simulink library "renewableCustom_lib"  (R2025b)
settings: Solver=VariableStepAuto  StartTime=0.0  StopTime=10.0  RelTol=1e-3
undefined symbols (not defined in the file or in its folder): alpha, Base, D, Kd, Kp, Kt, Ld, Lq, PVController, PVInverter, Rs, T, Ts
libraries: slpidlib x2, eeTransforms x2, simulink x2
settings Model: Creator=rajarshd  LastModifiedBy=rajarshd

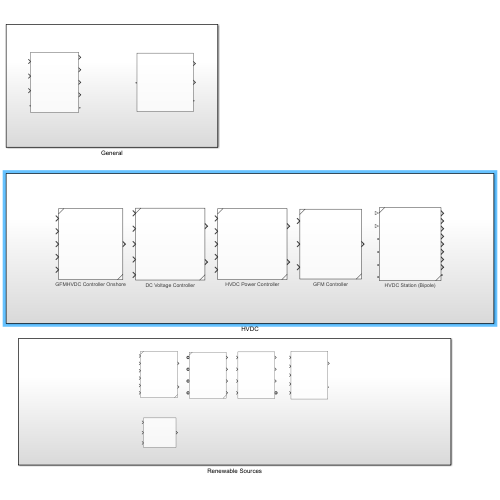
[thumbnail: Simulink's stored preview of the top-level diagram]
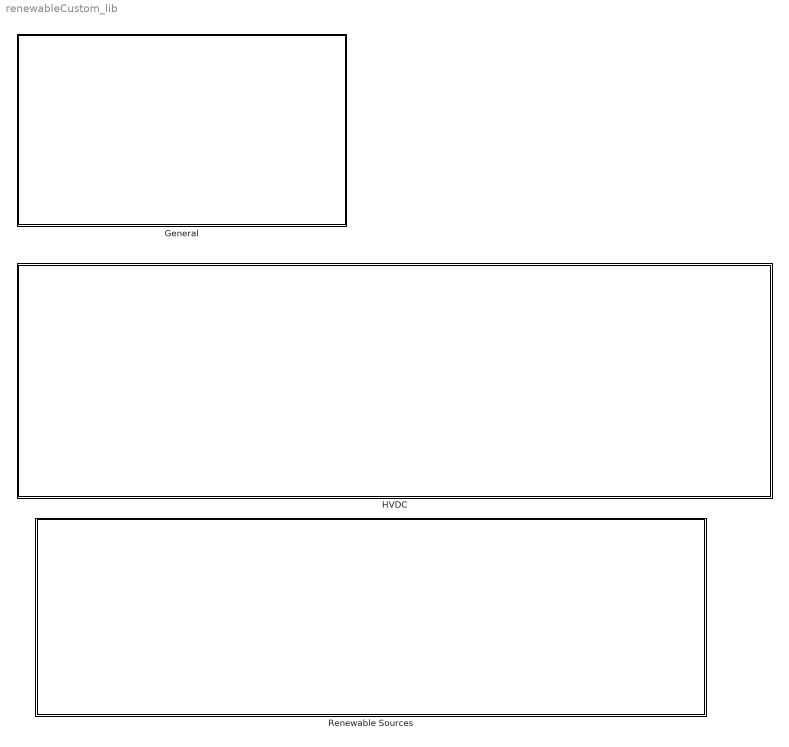
== system renewableCustom_lib ==
  General : Subsystem
  HVDC : Subsystem
  Renewable Sources : Subsystem

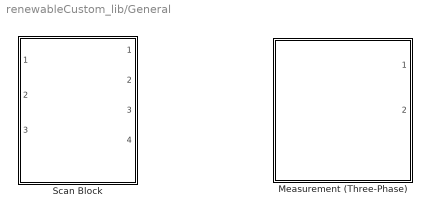
== system renewableCustom_lib/General ==
  Measurement (Three-Phase) : Subsystem  ReferencedSubsystem=MeasurementPLL  f=60  MVA=100e6  baseV=230e3
  Scan Block : Subsystem  ReferencedSubsystem=ScanBlockwithDC  F0=grid.frequency  Theta0=0  Kp_LF=100  Ki_LF=2000  Ts=5e-5  voltage=4.16e3  voltagedc=0  mva=0  Amplitude=0.01  Amplitude1=0  Amplitudedc=0  f=1:1:1e3  T=T  Tdis=5  Tend=10  VSelect=Equivalent Series Voltage (V)  Hold=Yes

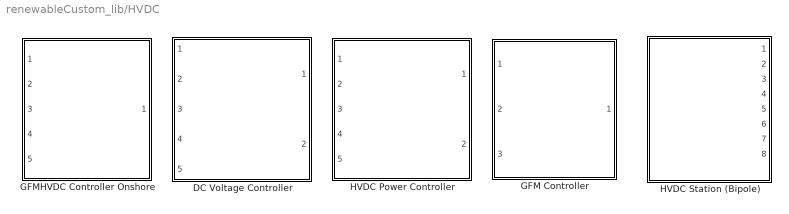
== system renewableCustom_lib/HVDC ==
  DC Voltage Controller : Subsystem  ReferencedSubsystem=DCVoltageControl  Kppll=100  Kipll=2000  frequency=60  initialPhase=0  sampleTime=-1  Kpicd=1.5  Kiicd=250  Kdicd=0  Kpicq=2  Kiicq=300  Kdicq=0  Kpv=20  Kiv=1  Kdv=0  L=5e-3  iMax=1.2  zBase=1.1  mVAbase=100e6  VdcBase=400e3
  GFM Controller : Subsystem  ReferencedSubsystem=WFController  Kpv=0  Kiv=0  Kpicd=0  Kiicd=0  Kpicq=0  Kiicq=0  mVAbase=0  frequency=0  zBase=0  iMax=0  L=0  Kv=0
  GFMHVDC Controller Onshore : Subsystem  ReferencedSubsystem=GFMHVDCControllerOnshore  D=10  J=0  frequency1=60  Pref=0  kc=0  Kq=0.1  VdRef=0  Imax1=1.2  l=5e-3  Kpv=5  Kiv=1  Vdc=0  Kpi=1.5  Kii=250
  HVDC Power Controller : Subsystem  ReferencedSubsystem=HVDCPowerControl  Kppll=PLL.Kp_pll  Kipll=PLL.Ki_pll  frequency=Grid.frequency  initialPhase=0  sampleTime=-1  Kpicd=PVController.Kp_ic  Kiicd=PVController.Ki_ic  Kdicd=0  Kpicq=PVController.Kp_ic  Kiicq=PVController.Ki_ic  Kdicq=0  Kpv=3.5  Kiv=10  Kdv=0.0  L=PVInverter.L*10  iMax=PVInverter.I_max_pu  zBase=Base.z_base  mVAbase=Base.MVA_base_new  VdcBase=PVController.Vdc_base
  HVDC Station (Bipole) : Subsystem  ReferencedSubsystem=HVDCSTATION  c=0  vc=0  L=0  VRated=0  SRated=0  t=0  Ts=0

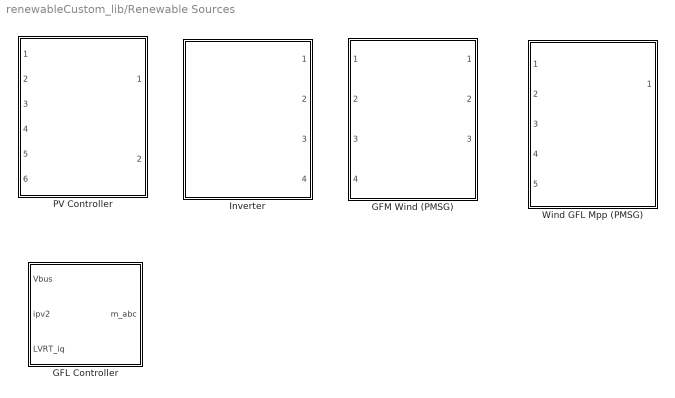
== system renewableCustom_lib/Renewable Sources ==
  GFL Controller : Subsystem  mask{Vref=1, fref=60, Pref=3e6, Qref=1e4, mp=1e-2, mv=2, P=Real power, MVA=5e7, zbase=2, L=3e-3, Imax=1.2, Td=3e-3, Kpic=2, Kiic=250, Kd=PVController.Kd}
      mask prompts: Vref "Voltage reference (PU)"; fref "Frequency reference (Hz)"; Pref "Real power reference (PU)"; Qref "Reactive power reference (PU)"; mp "Real power droop cofficient"; mv "Reactive power droop cofficient"; P "Priority mode"; MVA "Base Power (V*A)"; zbase "Base Impedance (Ohm)"; L "Filter Inductance (H)"; Imax "Inverter current limit (pu)"; Td "Sensor time delay (s)"; Kpic "Proportional gain"; Kiic "Integral gain"; Kd "Derevative gain"
      mask TypeOptions P: Real power  | Reactive power
      mask DialogControl Container4 Prompt: General
      mask DialogControl Container5 Prompt: Current Controller
      mask Display: image('$imagefile'); % Use "Edit Image" on toolstrip to change.
  GFM Wind (PMSG) : Subsystem  ReferencedSubsystem=gfmWind  Control=VSM Using DC Link Voltage  V_ref=V_ref  Q_ref=Q_ref  Kq=Kq_dc  Kt=Kt  KqI=Kq  Kp=Kp  Kd=Kd  Kj=Kj  H=H  D=D  Vd_ref=0  frequency1=0  frequency=0  Spref=Curtailed Power Operation  tstart=0  Vslope=0  Pstart=0  Pslope=0  x_vir=0  x_vir1=0  r_vir1=0  Imax1=0  Imax=0  r_vir=0  Kpq_mpp=Lq*alpha  Kpd_mpp=Ld*alpha  Kiq_mpp=Rs*alpha  Kid_mpp=Rs*alpha  Kpq=Lq*alpha  Kpd=Ld*alpha  Kiq=Rs*alpha  Kid=Rs*alpha  Kp_dc_sm=Kp_dc_sm  Ki_dc_sm=Ki_dc_sm  wt1=0  rt1=0  pitch1=0  cp1=0  airDensity1=0  TSR1=0  Radius1=0  wt=0.01  rt=0.01  pitch=pitch  cp=cp  airDensity=airDensity  Radius=turbineRadius  TSR=TSR  Inertia1=0  Inertia=0  psim1=0  p1=0  Rs1=0  Lq1=0  Ld1=0  Ld=Ld  Lq=Lq  Rs=Rs  p=p  psim=psim
  Inverter : Subsystem  ReferencedSubsystem=PVInverterGFL  c=1e-6 F  g=0 1/Ohm  vc_priority=None  vc_specify=on  vc=8000 V  Pfixed=1 W  L=5e-3 H  R=1e-3 Ohm  VRated=4.16e3  SRated=1e8
  PV Controller : Subsystem  ReferencedSubsystem=PVcontroller  L=5e-3  frequency=60  iMax=1.2  zBase=1.1  mVAbase=100e6  VdcBase=1e3  sampleTime=-1  Choice=Incremental conductance (INC)  Vdc=750  delV=10  tSettling=1e-3  Kppll=200  Kipll=1000  initialPhase=0  Kpv=1  Kiv=20  Kdv=0  Kpicd=2  Kiicd=250  Kdicd=0  Kpicq=2  Kiicq=250  Kdicq=0
  Wind GFL Mpp (PMSG) : Subsystem  ReferencedSubsystem=WindGFLMpp  p=0  psim=0  Rs=0  Ld=0  Lq=0  Kdip_sm=0  Kdii_sm=0  Kqip_sm=0  Kqii_sm=0  airDensity=0  turbineRadius=0  pitch=0  TSR=0  cp=0  wt=0  rt=0  Inertia=0  Kp_dc=0  Ki_dc=0  Kdpi_g=0  Kdii_g=0  Kqpi_g=0  Kqii_g=0  blk=Enabled  slop=0  tst=0

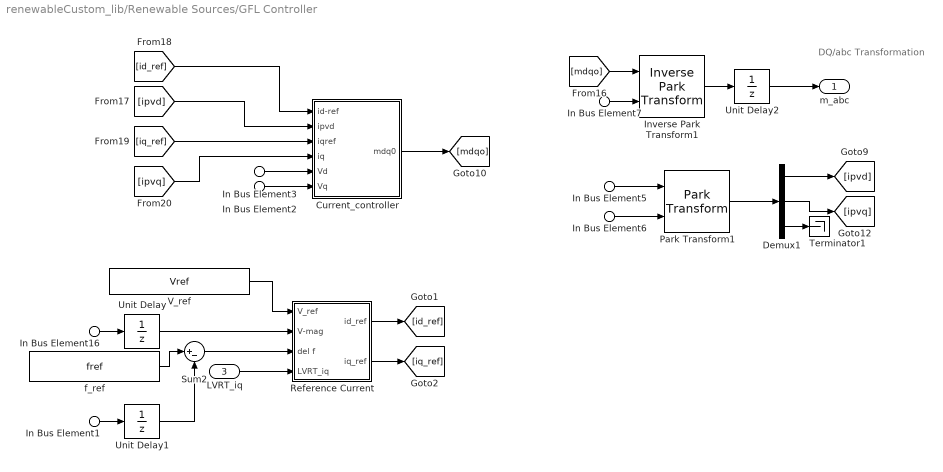
== system renewableCustom_lib/Renewable Sources/GFL Controller ==
  note: DQ/abc Transformation
  In Bus Element3 : Inport  PortName=Vbus  Element=Vd
  In Bus Element16 : Inport  PortName=Vbus  Element=Vd
  In Bus Element2 : Inport  PortName=Vbus  Element=Vq
  In Bus Element6 : Inport  PortName=Vbus  Element=Theta
  In Bus Element7 : Inport  PortName=Vbus  Element=Theta
  In Bus Element1 : Inport  PortName=Vbus  Element=w
  In Bus Element5 : Inport  Port=2  PortName=ipv2  Element=1
  LVRT_iq : Inport  Port=3
  Current_controller : Subsystem
  Demux1 : Demux  Outputs=3
  Inverse Park Transform1 : eeTransforms/Inverse Park Transform  AxisAlignment=Q-axis  PowerInvariant=off
  Park Transform1 : eeTransforms/Park Transform  AxisAlignment=Q-axis  PowerInvariant=off
  Reference Current : Subsystem
  Sum2 : Sum  Inputs=|+-
  Terminator1 : Terminator
  Unit Delay : UnitDelay  SampleTime=Td  HasFrameUpgradeWarning=on
  Unit Delay1 : UnitDelay  SampleTime=Td  HasFrameUpgradeWarning=on
  Unit Delay2 : UnitDelay  SampleTime=Ts  HasFrameUpgradeWarning=on
  V_ref : Constant  Value=Vref
  f_ref : Constant  Value=fref
  m_abc : Outport
  wires:
  In Bus Element2/1 -> Current_controller/6(Vq)
  Current_controller/1(mdq0) -> [mdqo]
  Inverse Park Transform1/1 -> Unit Delay2/1
  Demux1/2 -> [ipvq]
  Unit Delay2/1 -> m_abc/1
  Demux1/1 -> [ipvd]
  Demux1/3 -> Terminator1/1
  [mdqo] -> Inverse Park Transform1/1
  Park Transform1/1 -> Demux1/1
  [id_ref] -> Current_controller/1(id-ref)
  In Bus Element3/1 -> Current_controller/5(Vd)
  [iq_ref] -> Current_controller/3(iqref)
  [ipvq] -> Current_controller/4(iq)
  In Bus Element6/1 -> Park Transform1/2
  In Bus Element7/1 -> Inverse Park Transform1/2
  [ipvd] -> Current_controller/2(ipvd)
  In Bus Element5/1 -> Park Transform1/1
  f_ref/1 -> Sum2/1
  V_ref/1 -> Reference Current/1(V_ref)
  In Bus Element16/1 -> Unit Delay/1
  LVRT_iq/1 -> Reference Current/4(LVRT_iq)
  Sum2/1 -> Reference Current/3(del f)
  Reference Current/2(iq_ref) -> [iq_ref]
  Reference Current/1(id_ref) -> [id_ref]
  In Bus Element1/1 -> Unit Delay1/1
  Unit Delay1/1 -> Sum2/2
  Unit Delay/1 -> Reference Current/2(V-mag)

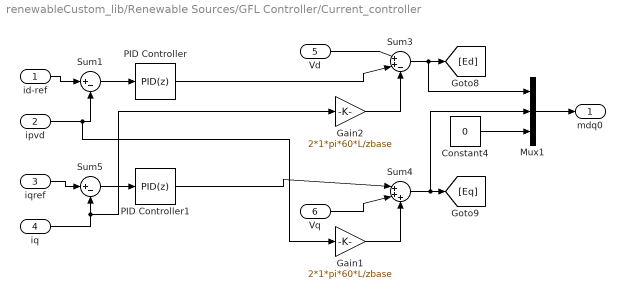
== system renewableCustom_lib/Renewable Sources/GFL Controller/Current_controller ==
  id-ref : Inport
  ipvd : Inport  Port=2
  iqref : Inport  Port=3
  iq : Inport  Port=4
  Vd : Inport  Port=5
  Vq : Inport  Port=6
  Constant4 : Constant  Value=0
  Gain1 : Gain  Gain=2*1*pi*60*L/zbase
  Gain2 : Gain  Gain=2*1*pi*60*L/zbase
  Mux1 : Mux  Inputs=3
  PID Controller : slpidlib/PID Controller  Controller=PID  Form=Parallel  TimeDomain=Discrete-time  UseExternalTs=off  SampleTime=-1  IntegratorMethod=Forward Euler  FilterMethod=Forward Euler  ControllerParametersSource=internal  P=Kpic  I=Kiic  UseKiTs=off  D=Kd  UseExternalDerivativeSource=off  N=100  UseFilter=on  TunerSelectOption=Transfer Function Based (PID Tuner App)  InitialConditionSource=internal  InitialConditionForIntegrator=0  InitialConditionForFilter=0  DifferentiatorICPrevScaledInput=0  ExternalReset=none  TrackingMode=off  Kt=1  LimitOutput=off  SatLimitsSource=internal  UpperSaturationLimit=inf  LowerSaturationLimit=-inf  LinearizeAsGain=on  AntiWindupMode=none  Kb=1  LimitIntegrator=off  UpperIntegratorSaturationLimit=inf  LowerIntegratorSaturationLimit=-inf  POutMin=[]  POutMax=[]  IOutMin=[]  IOutMax=[]  DOutMin=[]  DOutMax=[]  NOutMin=[]  NOutMax=[]  SumOutMin=[]  SumOutMax=[]  SaturationOutMin=[]  SaturationOutMax=[]  PParamMin=[]  PParamMax=[]  IParamMin=[]  IParamMax=[]  DParamMin=[]  DParamMax=[]  NParamMin=[]  NParamMax=[]  KbParamMin=[]  KbParamMax=[]  KtParamMin=[]  KtParamMax=[]  KbOutMin=[]  KbOutMax=[]  KtOutMin=[]  KtOutMax=[]  IntegratorOutMin=[]  IntegratorOutMax=[]  FilterOutMin=[]  FilterOutMax=[]  SumI1OutMin=[]  SumI1OutMax=[]  SumI2OutMin=[]  SumI2OutMax=[]  SumI3OutMin=[]  SumI3OutMax=[]  SumI4OutMin=[]  SumI4OutMax=[]  SumDOutMin=[]  SumDOutMax=[]  DifferentiatorOutMin=[]  DifferentiatorOutMax=[]  FilterDiffOutCoefMin=[]  FilterDiffOutCoefMax=[]  ReciprocalOutMin=[]  ReciprocalOutMax=[]  SumDenOutMin=[]  SumDenOutMax=[]  SumNumOutMin=[]  SumNumOutMax=[]  DivideOutMin=[]  DivideOutMax=[]  UdiffTsProdOutMin=[]  UdiffTsProdOutMax=[]  NTsProdOutMin=[]  NTsProdOutMax=[]  UintegralTsProdOutMin=[]  UintegralTsProdOutMax=[]  UngainTsProdOutMin=[]  UngainTsProdOutMax=[]  ClampingZeroOutDataTypeStr=Inherit: Inherit via back propagation  ClampingZeroOutMin=[]  ClampingZeroOutMax=[]  FilterDenConstantOutDataTypeStr=Inherit: Inherit via back propagation  FilterDenConstantOutMin=[]  FilterDenConstantOutMax=[]  PCopyOutDataTypeStr=Inherit: Inherit via back propagation  PCopyOutMin=[]  PCopyOutMax=[]  NCopyOutDataTypeStr=Inherit: Inherit via back propagation  NCopyOutMin=[]  NCopyOutMax=[]  IntegratorContinuousStateAttributes=''  IntegratorStateMustResolveToSignalObject=off  IntegratorRTWStateStorageClass=Auto  FilterContinuousStateAttributes=''  FilterStateMustResolveToSignalObject=off  FilterRTWStateStorageClass=Auto  ParallelPVariant=InternalParameters  IdealPVariant=Disabled  IVariant=InternalParameters  DVariant=InternalParameters  IntegratorVariant=Discrete  SatVariant=Disabled  AWVariant=Passthrough  PCopyVariant=Disabled  TRVariant=Disabled  FdbkBlocksVariant=Forward  IdealPFdbkVariant=Disabled  SatFdbkVariant=Disabled  DerivativeFilterVariant=ForwardEulerFilter  NVariant=InternalParameters  NCopyVariant=Disabled  FilterICVariant=InternalICsFilter  IntegratorICVariant=InternalICs  ExternalResetVariant=Disabled  TRSumVariant=Passthrough  SumFdbkVariant=Disabled  SumVariant=Sum_PID  TsampFilterVariant=InternalTs  TsampNgainVariant=Passthrough  TsampIntegralVariant=Disabled_SignalSpec  ExternalSaturationOutDataTypeStr=Inherit: Same as second input  DerivativeSourceVariant=ErrorSignal  PreIntVariant=InternalPreInt
  PID Controller1 : slpidlib/PID Controller  Controller=PID  Form=Parallel  TimeDomain=Discrete-time  UseExternalTs=off  SampleTime=-1  IntegratorMethod=Forward Euler  FilterMethod=Forward Euler  ControllerParametersSource=internal  P=Kpic  I=Kiic  UseKiTs=off  D=Kd  UseExternalDerivativeSource=off  N=100  UseFilter=on  TunerSelectOption=Transfer Function Based (PID Tuner App)  InitialConditionSource=internal  InitialConditionForIntegrator=0  InitialConditionForFilter=0  DifferentiatorICPrevScaledInput=0  ExternalReset=none  TrackingMode=off  Kt=1  LimitOutput=off  SatLimitsSource=internal  UpperSaturationLimit=inf  LowerSaturationLimit=-inf  LinearizeAsGain=on  AntiWindupMode=none  Kb=1  LimitIntegrator=off  UpperIntegratorSaturationLimit=inf  LowerIntegratorSaturationLimit=-inf  POutMin=[]  POutMax=[]  IOutMin=[]  IOutMax=[]  DOutMin=[]  DOutMax=[]  NOutMin=[]  NOutMax=[]  SumOutMin=[]  SumOutMax=[]  SaturationOutMin=[]  SaturationOutMax=[]  PParamMin=[]  PParamMax=[]  IParamMin=[]  IParamMax=[]  DParamMin=[]  DParamMax=[]  NParamMin=[]  NParamMax=[]  KbParamMin=[]  KbParamMax=[]  KtParamMin=[]  KtParamMax=[]  KbOutMin=[]  KbOutMax=[]  KtOutMin=[]  KtOutMax=[]  IntegratorOutMin=[]  IntegratorOutMax=[]  FilterOutMin=[]  FilterOutMax=[]  SumI1OutMin=[]  SumI1OutMax=[]  SumI2OutMin=[]  SumI2OutMax=[]  SumI3OutMin=[]  SumI3OutMax=[]  SumI4OutMin=[]  SumI4OutMax=[]  SumDOutMin=[]  SumDOutMax=[]  DifferentiatorOutMin=[]  DifferentiatorOutMax=[]  FilterDiffOutCoefMin=[]  FilterDiffOutCoefMax=[]  ReciprocalOutMin=[]  ReciprocalOutMax=[]  SumDenOutMin=[]  SumDenOutMax=[]  SumNumOutMin=[]  SumNumOutMax=[]  DivideOutMin=[]  DivideOutMax=[]  UdiffTsProdOutMin=[]  UdiffTsProdOutMax=[]  NTsProdOutMin=[]  NTsProdOutMax=[]  UintegralTsProdOutMin=[]  UintegralTsProdOutMax=[]  UngainTsProdOutMin=[]  UngainTsProdOutMax=[]  ClampingZeroOutDataTypeStr=Inherit: Inherit via back propagation  ClampingZeroOutMin=[]  ClampingZeroOutMax=[]  FilterDenConstantOutDataTypeStr=Inherit: Inherit via back propagation  FilterDenConstantOutMin=[]  FilterDenConstantOutMax=[]  PCopyOutDataTypeStr=Inherit: Inherit via back propagation  PCopyOutMin=[]  PCopyOutMax=[]  NCopyOutDataTypeStr=Inherit: Inherit via back propagation  NCopyOutMin=[]  NCopyOutMax=[]  IntegratorContinuousStateAttributes=''  IntegratorStateMustResolveToSignalObject=off  IntegratorRTWStateStorageClass=Auto  FilterContinuousStateAttributes=''  FilterStateMustResolveToSignalObject=off  FilterRTWStateStorageClass=Auto  ParallelPVariant=InternalParameters  IdealPVariant=Disabled  IVariant=InternalParameters  DVariant=InternalParameters  IntegratorVariant=Discrete  SatVariant=Disabled  AWVariant=Passthrough  PCopyVariant=Disabled  TRVariant=Disabled  FdbkBlocksVariant=Forward  IdealPFdbkVariant=Disabled  SatFdbkVariant=Disabled  DerivativeFilterVariant=ForwardEulerFilter  NVariant=InternalParameters  NCopyVariant=Disabled  FilterICVariant=InternalICsFilter  IntegratorICVariant=InternalICs  ExternalResetVariant=Disabled  TRSumVariant=Passthrough  SumFdbkVariant=Disabled  SumVariant=Sum_PID  TsampFilterVariant=InternalTs  TsampNgainVariant=Passthrough  TsampIntegralVariant=Disabled_SignalSpec  ExternalSaturationOutDataTypeStr=Inherit: Same as second input  DerivativeSourceVariant=ErrorSignal  PreIntVariant=InternalPreInt
  Sum1 : Sum  Inputs=|+-
  Sum3 : Sum  Inputs=|++-
  Sum4 : Sum  Inputs=|+++
  Sum5 : Sum  Inputs=|+-
  mdq0 : Outport
  wires:
  PID Controller/1 -> Sum3/2
  Sum3/1 -> Mux1/1, [Ed]
  Gain2/1 -> Sum3/3
  ipvd/1 -> Gain1/1, Sum1/2
  id-ref/1 -> Sum1/1
  Gain1/1 -> Sum4/3
  Vq/1 -> Sum4/2
  iq/1 -> Gain2/1, Sum5/2
  Sum1/1 -> PID Controller/1
  Vd/1 -> Sum3/1
  Constant4/1 -> Mux1/3
  Sum5/1 -> PID Controller1/1
  iqref/1 -> Sum5/1
  PID Controller1/1 -> Sum4/1
  Sum4/1 -> Mux1/2, [Eq]
  Mux1/1 -> mdq0/1

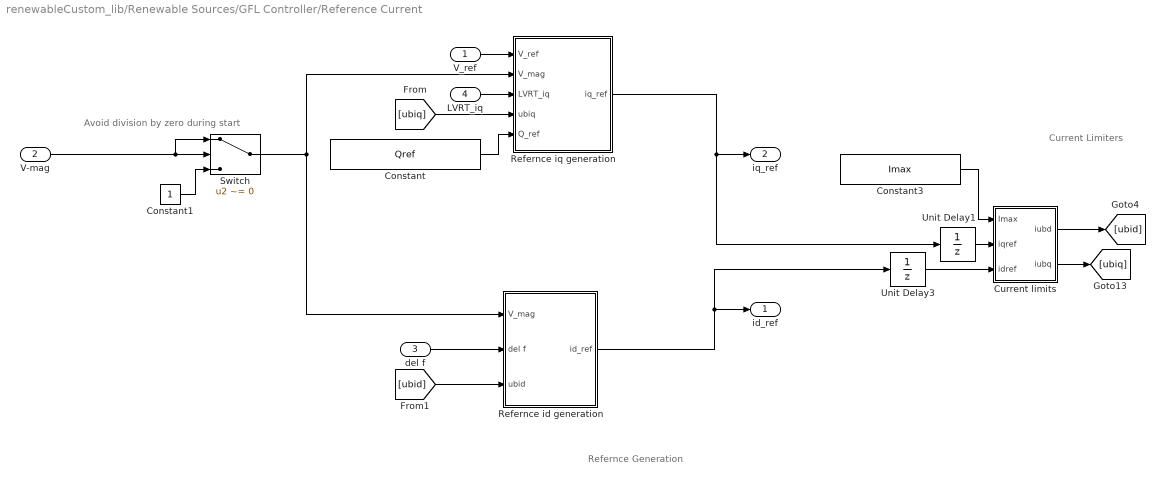
== system renewableCustom_lib/Renewable Sources/GFL Controller/Reference Current ==
  note: Refernce Generation
  note: Current Limiters
  note: Avoid division by zero during start
  V_ref : Inport
  V-mag : Inport  Port=2
  del f : Inport  Port=3
  LVRT_iq : Inport  Port=4
  Constant : Constant  Value=Qref
  Constant1 : Constant
  Constant3 : Constant  Value=Imax
  Current limits : Subsystem
  Refernce id generation : Subsystem
  Refernce iq generation : Subsystem
  Switch : Switch  Criteria=u2 ~= 0  SaturateOnIntegerOverflow=off  InputSameDT=off
  Unit Delay1 : UnitDelay  SampleTime=Ts  HasFrameUpgradeWarning=on
  Unit Delay3 : UnitDelay  SampleTime=Ts  HasFrameUpgradeWarning=on
  id_ref : Outport
  iq_ref : Outport  Port=2
  wires:
  Current limits/1(iubd) -> [ubid]
  Unit Delay1/1 -> Current limits/2(iqref)
  Current limits/2(iubq) -> [ubiq]
  Unit Delay3/1 -> Current limits/3(idref)
  Constant3/1 -> Current limits/1(Imax)
  Refernce id generation/1(id_ref) -> id_ref/1, Unit Delay3/1
  del f/1 -> Refernce id generation/2(del f)
  V_ref/1 -> Refernce iq generation/1(V_ref)
  Refernce iq generation/1(iq_ref) -> Unit Delay1/1, iq_ref/1
  LVRT_iq/1 -> Refernce iq generation/3(LVRT_iq)
  [ubiq] -> Refernce iq generation/4(ubiq)
  [ubid] -> Refernce id generation/3(ubid)
  V-mag/1 -> Switch/1, Switch/2
  Switch/1 -> Refernce id generation/1(V_mag), Refernce iq generation/2(V_mag)
  Constant1/1 -> Switch/3
  Constant/1 -> Refernce iq generation/5(Q_ref)

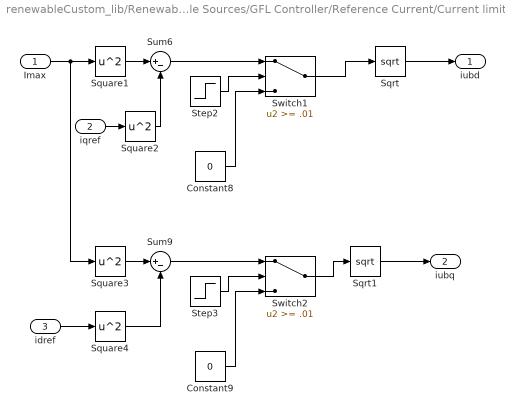
== system renewableCustom_lib/Renewable Sources/GFL Controller/Reference Current/Current limits ==
  Imax : Inport
  iqref : Inport  Port=2
  idref : Inport  Port=3
  Constant8 : Constant  Value=0
  Constant9 : Constant  Value=0
  Sqrt : Sqrt
  Sqrt1 : Sqrt
  Square{1..4} (4 alike) : Math  Operator=square
  Step2 : Step  Time=0.01  SampleTime=Ts
  Step3 : Step  Time=0.01  SampleTime=Ts
  Sum6 : Sum  Inputs=|+-
  Sum9 : Sum  Inputs=|+-
  Switch1 : Switch  Threshold=.01  SaturateOnIntegerOverflow=off  InputSameDT=off
  Switch2 : Switch  Threshold=.01  SaturateOnIntegerOverflow=off  InputSameDT=off
  iubd : Outport
  iubq : Outport  Port=2
  wires:
  Sum9/1 -> Switch2/1
  Step3/1 -> Switch2/2
  Step2/1 -> Switch1/2
  Switch2/1 -> Sqrt1/1
  Square1/1 -> Sum6/1
  Switch1/1 -> Sqrt/1
  iqref/1 -> Square2/1
  Square3/1 -> Sum9/1
  Sum6/1 -> Switch1/1
  Square2/1 -> Sum6/2
  Constant8/1 -> Switch1/3
  Square4/1 -> Sum9/2
  Constant9/1 -> Switch2/3
  Sqrt/1 -> iubd/1
  Imax/1 -> Square3/1, Square1/1
  Sqrt1/1 -> iubq/1
  idref/1 -> Square4/1

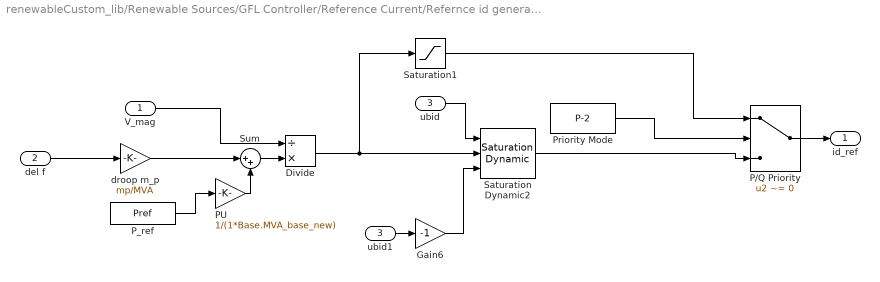
== system renewableCustom_lib/Renewable Sources/GFL Controller/Reference Current/Refernce id generation ==
  V_mag : Inport
  del f : Inport  Port=2
  ubid : Inport  Port=3
  Divide : Product  Inputs=/*
  Gain6 : Gain  Gain=-1
  P/Q Priority : Switch  Criteria=u2 ~= 0  SaturateOnIntegerOverflow=off  InputSameDT=off
  PU : Gain  Gain=1/(1*Base.MVA_base_new)
  P_ref : Constant  Value=Pref
  Priority Mode : Constant  Value=P-2
  Saturation Dynamic2 : simulink/Discontinuities/Saturation Dynamic  OutMin=[]  OutMax=[]  OutDataTypeStr=Inherit: Same as second input  OutDataType=fixdt(1, 16)  OutScaling=2^-10  DoSatur=off
  Saturation1 : Saturate  UpperLimit=Imax  LowerLimit=-Imax
  Sum : Sum  Inputs=|++
  droop m_p : Gain  Gain=mp/MVA
  ubid1 : InportShadow  Port=3
  id_ref : Outport
  wires:
  P_ref/1 -> PU/1
  droop m_p/1 -> Sum/1
  Sum/1 -> Divide/2
  ubid/1 -> Saturation Dynamic2/1
  Gain6/1 -> Saturation Dynamic2/3
  Saturation Dynamic2/1 -> P/Q Priority/3
  PU/1 -> Sum/2
  Priority Mode/1 -> P/Q Priority/2
  Saturation1/1 -> P/Q Priority/1
  ubid1/1 -> Gain6/1
  P/Q Priority/1 -> id_ref/1
  V_mag/1 -> Divide/1
  Divide/1 -> Saturation1/1, Saturation Dynamic2/2
  del f/1 -> droop m_p/1

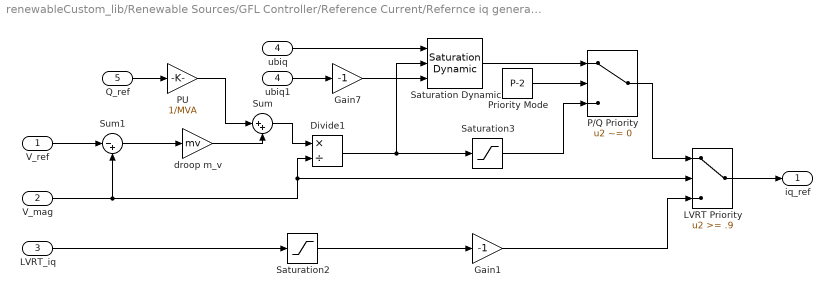
== system renewableCustom_lib/Renewable Sources/GFL Controller/Reference Current/Refernce iq generation ==
  V_ref : Inport
  V_mag : Inport  Port=2
  LVRT_iq : Inport  Port=3
  ubiq : Inport  Port=4
  Q_ref : Inport  Port=5
  Divide1 : Product  Inputs=*/
  Gain1 : Gain  Gain=-1
  Gain7 : Gain  Gain=-1
  LVRT Priority : Switch  Threshold=.9  SaturateOnIntegerOverflow=off  InputSameDT=off
  P/Q Priority : Switch  Criteria=u2 ~= 0  SaturateOnIntegerOverflow=off  InputSameDT=off
  PU : Gain  Gain=1/MVA
  Priority Mode : Constant  Value=P-2
  Saturation Dynamic : simulink/Discontinuities/Saturation Dynamic  OutMin=[]  OutMax=[]  OutDataTypeStr=Inherit: Same as second input  OutDataType=fixdt(1, 16)  OutScaling=2^-10  DoSatur=off
  Saturation2 : Saturate  UpperLimit=1  LowerLimit=-1
  Saturation3 : Saturate  UpperLimit=Imax  LowerLimit=-Imax
  Sum : Sum  Inputs=|++
  Sum1 : Sum  Inputs=|-+
  droop m_v : Gain  Gain=mv
  ubiq1 : InportShadow  Port=4
  iq_ref : Outport
  wires:
  LVRT Priority/1 -> iq_ref/1
  Sum1/1 -> droop m_v/1
  P/Q Priority/1 -> LVRT Priority/1
  Gain1/1 -> LVRT Priority/3
  ubiq/1 -> Saturation Dynamic/1
  Saturation2/1 -> Gain1/1
  Saturation3/1 -> P/Q Priority/3
  Priority Mode/1 -> P/Q Priority/2
  Divide1/1 -> Saturation Dynamic/2, Saturation3/1
  Saturation Dynamic/1 -> P/Q Priority/1
  Gain7/1 -> Saturation Dynamic/3
  V_ref/1 -> Sum1/1
  LVRT_iq/1 -> Saturation2/1
  V_mag/1 -> Sum1/2, LVRT Priority/2, Divide1/2
  ubiq1/1 -> Gain7/1
  droop m_v/1 -> Sum/2
  Sum/1 -> Divide1/1
  Q_ref/1 -> PU/1
  PU/1 -> Sum/1
